simulink model "test_temperatura_simulink"  (R2025a)
settings: Solver=VariableStepAuto  StartTime=0.0  StopTime=10.0  RelTol=1e-3
libraries: fuzblock x1
settings Model: Creator=Bremdows  LastModifiedBy=Bremdows

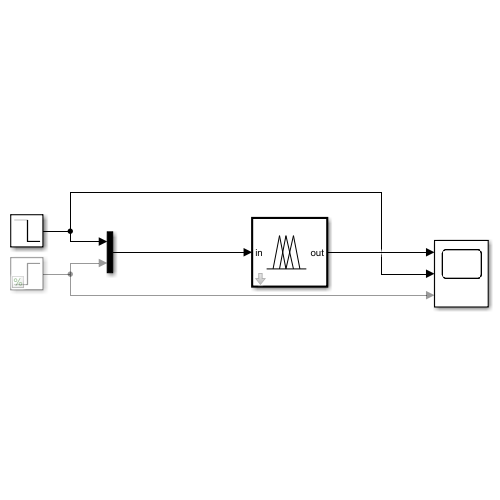
[thumbnail: Simulink's stored preview of the top-level diagram]
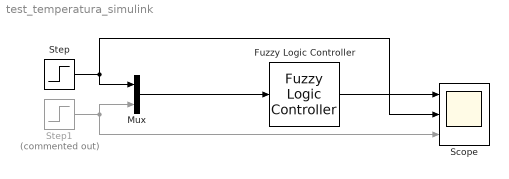
== system test_temperatura_simulink ==
  Fuzzy Logic Controller : fuzblock/Fuzzy Logic  Controller  FIS=testperatura  OutputSampleNumber=101  DataType=double  UseLookupTable=off  NumBreakpoints=10  FuzzifiedInputs=off  RuleFiringStrengths=off  RuleOutputs=off  AggregatedOutputs=off  SimulateUsing=Interpreted execution  OutOfRangeInputValueMessage=warning  NoRuleFiredMessage=warning  EmptyOutputFuzzySetMessage=warning
  Mux : Mux  Inputs=2
  Scope : Scope  NumInputPorts=3
      settings: ActiveDisplayYMinimum=-12.203  ActiveDisplayYMaximum=9.827
  Step : Step  Time=0  After=-10  SampleTime=0
  Step1 : Step  Commented=on  Time=0  After=5  SampleTime=0
  wires:
  Mux/1 -> Fuzzy Logic Controller/1
  Fuzzy Logic Controller/1 -> Scope/1
  Step/1 -> Scope/2, Mux/1
  Step1/1 -> Scope/3, Mux/2
